simulink model "final_obc"  (R2022a)
settings: Solver=VariableStepAuto  StartTime=0.0  StopTime=0.7  RelTol=1e-3
values from neighbouring files (symbols this model uses):
  ccControl_Kaw = 0    [final.mat]
  cvControl_Kaw = 1    [final.mat]
  Ki = 46    [final.mat]
  Kp = 0.22    [final.mat]
  Ts = 5e-06    [final.mat]
  Tsc = 0.0001    [final.mat]
libraries: fl_lib x18, nesl_utility x17, ee_lib x11, eeGeneralControl x6, slpidlib x4, spsPWMGeneratorDCDCLib x4, spsTHDLib x4, eeDcDcVoltageController x1, eePwmGenerator x1
(part 2 of 2)

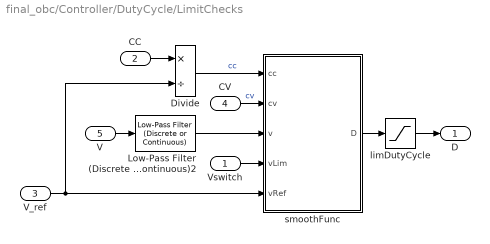
== system final_obc/Controller/DutyCycle/LimitChecks ==
  Vswitch : Inport
  CC : Inport  Port=2
  V_ref : Inport  Port=3
  CV : Inport  Port=4
  V : Inport  Port=5
  Divide : Product  Inputs=*/
  Low-Pass Filter (Discrete or Continuous)2 : eeGeneralControl/Low-Pass Filter (Discrete or Continuous)  K=1  T=1  B=inf  A=-inf  init_option=Inherited from block input  x0=0  Ts=0
  limDutyCycle : Saturate  UpperLimit=.99  LowerLimit=0.0001
  smoothFunc : MATLAB Function  TreatAsAtomicUnit=on
  D : Outport
  wires:
  V_ref/1 -> Divide/2, smoothFunc/5(vRef)
  CC/1 -> Divide/1
  limDutyCycle/1 -> D/1
  smoothFunc/1(D) -> limDutyCycle/1
  Divide/1 -> smoothFunc/1(cc)  "cc"
  V/1 -> Low-Pass Filter (Discrete or Continuous)2/1
  Vswitch/1 -> smoothFunc/4(vLim)
  CV/1 -> smoothFunc/2(cv)  "cv"
  Low-Pass Filter (Discrete or Continuous)2/1 -> smoothFunc/3(v)

== system final_obc/Controller/Feedback/SOCcheck ==
  SOC : Inport
  Constant3 : Constant  Value=0.9999
  Constant4 : Constant  Value=0
  MinMax : MinMax  Function=max  Inputs=2
  Subtract : Sum  Inputs=+-
  state : Outport
  wires:
  Constant4/1 -> MinMax/2
  Subtract/1 -> MinMax/1
  Constant3/1 -> Subtract/2
  MinMax/1 -> state/1
  SOC/1 -> Subtract/1

== matlab function final_obc/Controller/DutyCycle/LimitChecks/smoothFunc ==
  data: cc input; D output; cv input; v input; vLim input; vRef input
function D = Dsmooth(cc,cv,v,vLim,vRef)
    f=min(1,max(0,(v-vLim)/(vRef-vLim)));
    %f=max(1,max(0,(v-vLim)/(vRef-vLim)));
    D=cc*(1-f)+cv*f;
end
